simulink model "waffle_kin_sim_test"  (R2020a)
settings: Solver=FixedStepAuto  StartTime=0.0  StopTime=inf  FixedStep=0.01  RelTol=1e-3
undefined symbols (not defined in the file): Angular, Linear
libraries: robotlib x3

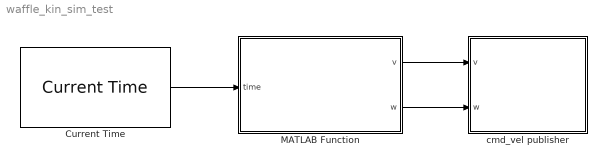
== system waffle_kin_sim_test ==
  Current Time : robotlib/Current Time  OutputFormat=double  SampleTime=-1  ModelName=waffle_kin_sim_test
  MATLAB Function : MATLAB Function  TreatAsAtomicUnit=on
  cmd_vel publisher : Subsystem  mask{simPublishRate=25}
      mask prompts: simPublishRate "Publishing rate [Hz]"
  wires:
  Current Time/1 -> MATLAB Function/1(time)
  MATLAB Function/1(v) -> cmd_vel publisher/1(v)
  MATLAB Function/2(w) -> cmd_vel publisher/2(w)

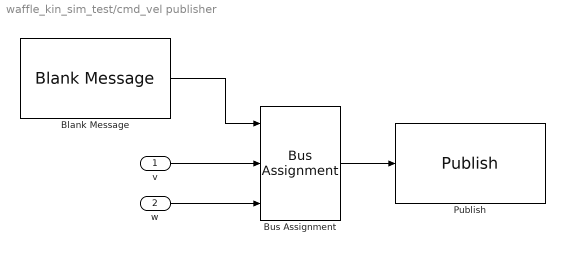
== system waffle_kin_sim_test/cmd_vel publisher ==
  v : Inport  SampleTime=1/simPublishRate
  w : Inport  Port=2  SampleTime=1/simPublishRate
  Blank Message : robotlib/Blank Message  messageClass=Message  entityType=geometry_msgs/Twist  messageType=geometry_msgs/Twist  SampleTime=1/simPublishRate
  Bus Assignment : BusAssignment  AssignedSignals=Linear.X,Angular.Z
  Publish : robotlib/Publish  topicSource=Specify your own  topic=/cmd_vel  messageType=geometry_msgs/Twist  messageQueueLength=1
  wires:
  Bus Assignment/1 -> Publish/1
  Blank Message/1 -> Bus Assignment/1
  v/1 -> Bus Assignment/2
  w/1 -> Bus Assignment/3

== matlab function waffle_kin_sim_test/MATLAB Function ==
function [v,w] = command_generator(time)

if (time<=10)
    v = 0.2;
    w = 0.0;
elseif (time<=20)
    v = 0.0;
    w = 90*pi/180/10;
elseif (time<=30)
    v = 0.2;
    w = 0.0;
elseif (time<=40)
    v = 0.0;
    w = 90*pi/180/10;
elseif (time<=50)
    v = 0.2;
    w = 0.0;
elseif (time<=60)
    v = 0.0;
    w = 90*pi/180/10;
elseif (time<=70)
    v = 0.2;
    w = 0.0;
else
    v = 0.0;
    w = 0.0;
end
